simulink model "Task3_2"  (R2020b)
settings: Solver=VariableStepAuto  StartTime=0.0  StopTime=90.0  RelTol=1e-3
values from neighbouring files (symbols this model uses):
  Ct = c0 + c1.*lambda + c2*lambda.^2    [Code2021_Jo_Saleh.m]    (also in ExeRet21.m.m)
  J = H * 2 * Sb / wm^2    (= 9574851.8542)    [Code2021_Jo_Saleh.m]    (also in ExeRet21.m.m)
  p = 180    [Code2021_Jo_Saleh.m]    (also in ExeRet21.m.m)
  r = 50    [Code2021_Jo_Saleh.m]    (also in ExeRet21.m.m)
  rho = 1.225    [Code2021_Jo_Saleh.m]    (also in ExeRet21.m.m)
  Te = 0:1e3:Te_rated    [Code2021_Jo_Saleh.m]    (also in ExeRet21.m.m)
  Vw_3 = 10    [Code2021_Jo_Saleh.m]    (also in ExeRet21.m.m)
  we_opt = p / 2 * wm_opt    (= 120.6)    [Code2021_Jo_Saleh.m]    (also in ExeRet21.m.m)
settings Model: Creator=Tomo  LastModifiedBy=Tomo

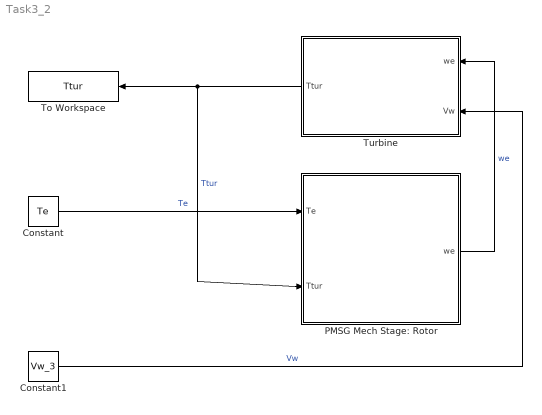
== system Task3_2 ==
  Constant : Constant  Value=Te
  Constant1 : Constant  Value=Vw_3
  PMSG Mech Stage: Rotor : Subsystem
  To Workspace : ToWorkspace  VariableName=Ttur  SampleTime=-1
  Turbine : Subsystem
  wires:
  Constant/1 -> PMSG Mech Stage: Rotor/1(Te)  "Te"
  PMSG Mech Stage: Rotor/1(we) -> Turbine/1(we)  "we"
  Turbine/1(Ttur) -> PMSG Mech Stage: Rotor/2(Ttur), To Workspace/1  "Ttur"
  Constant1/1 -> Turbine/2(Vw)  "Vw"

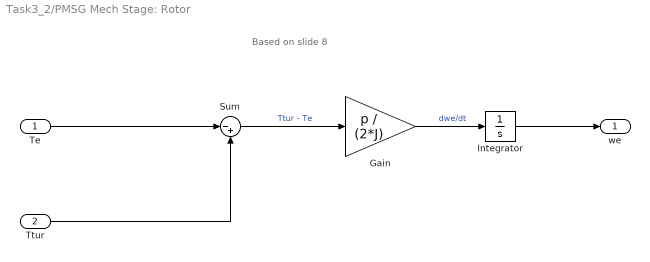
== system Task3_2/PMSG Mech Stage: Rotor ==
  note: Based on slide 8
  Te : Inport
  Ttur : Inport  Port=2
  Gain : Gain  Gain=p / (2*J)
  Integrator : Integrator  InitialCondition=we_opt
  Sum : Sum  Inputs=|-+
  we : Outport
  wires:
  Gain/1 -> Integrator/1  "dwe/dt"
  Integrator/1 -> we/1
  Sum/1 -> Gain/1  "Ttur - Te"
  Te/1 -> Sum/1
  Ttur/1 -> Sum/2

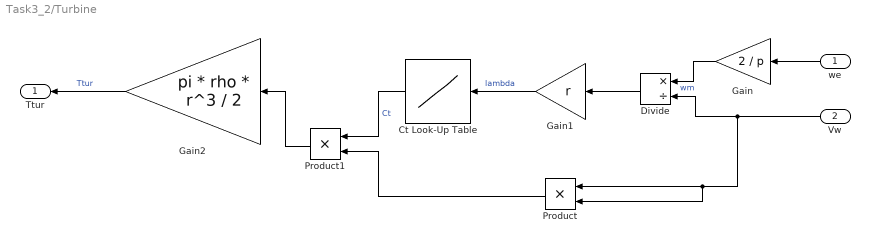
== system Task3_2/Turbine ==
  we : Inport
  Vw : Inport  Port=2
  Ct Look-Up Table : Lookup_n-D  NumberOfTableDimensions=1  BreakpointsForDimension1=[0:1e-2:20]  Table=Ct  InternalRulePriority=Speed  RndMeth=Simplest  InputSameDT=on
  Divide : Product  Inputs=*/
  Gain : Gain  Gain=2 / p
  Gain1 : Gain  Gain=r
  Gain2 : Gain  Gain=pi * rho * r^3 / 2
  Product : Product
  Product1 : Product
  Ttur : Outport
  wires:
  we/1 -> Gain/1
  Gain2/1 -> Ttur/1  "Ttur"
  Ct Look-Up Table/1 -> Product1/1  "Ct"
  Gain/1 -> Divide/1  "wm"
  Gain1/1 -> Ct Look-Up Table/1  "lambda"
  Vw/1 -> Product/2, Product/1, Divide/2
  Divide/1 -> Gain1/1
  Product/1 -> Product1/2
  Product1/1 -> Gain2/1
